simulink model "Engine_GT_RT_Model_Test"  (R2016b)
settings: Solver=VariableStepAuto  StartTime=0.0  StopTime=10.0  RelTol=1e-3
libraries: gtlink2017rt x1
settings Model: Creator=r03schne  LastModifiedBy=r03schne

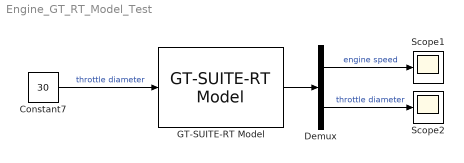
== system Engine_GT_RT_Model_Test ==
  Constant7 : Constant  Value=30
  Demux : Demux  Outputs=2
  GT-SUITE-RT Model : gtlink2017rt/GT-SUITE-RT Model  gti_fname=1cylDI-final  gti_dur=SIMULINK  gti_msg=No runtime messages  gti_dt=0.001  gti_ni=1  gti_no=2  gti_parnam='ign'  gti_parval='ign'  gti_cylnam='ign'  gti_nrtpr=-1
      settings: AttributesFormatString=(%<gti_fname>.dat)
  Scope1 : Scope
  Scope2 : Scope
  wires:
  Constant7/1 -> GT-SUITE-RT Model/1  "throttle diameter"
  GT-SUITE-RT Model/1 -> Demux/1
  Demux/1 -> Scope1/1  "engine speed"
  Demux/2 -> Scope2/1  "throttle diameter"
